simulink model "MoreElectricAircraftEMSHIL"  (R2023a)
settings: Solver=FixedStepAuto  StartTime=0.0  StopTime=350  RelTol=1e-3  EnableMultiTasking=on
PreLoadFcn:
  | Ts=100e-6;
InitFcn:
  | Ts=100e-6;
undefined symbols (not defined in the file): DiscIntNeverNeededParam, getfullname, IO682, Ion, Lithium
libraries: spsCurrentMeasurementLib x21, spsSeriesRLCBranchLib x19, spsVoltageMeasurementLib x19, speedgoatlib_IO682 x14, spsDiodeLib x10, spsControlledCurrentSourceLib x8, simulink x8, spsControlledVoltageSourceLib x7, spsIdealSwitchLib x6, spsThreePhaseParallelRLCLoadLib x1, spsPLL3phLib x1, spsThreePhaseVIMeasurementLib x1
(part 1 of 4)
settings Model: Creator=The MathWorks, Inc.  LastModifiedBy=steve.liu
settings SolverCC: ConcurrentTasks=on  AlgebraicLoopSolver=TrustRegion  PositivePriorityOrder=on  AutoInsertRateTranBlk=on
settings DataIOCC: LimitDataPoints=on  SaveFormat=Array  ReturnWorkspaceOutputs=off
settings OptimizationCC: BlockReduction=off  OptimizeBlockIOStorage=off  ReuseModelBlockBuffer=off  ExpressionDepthLimit=2147483647  EfficientMapNaN2IntZero=off
settings DebuggingCC: UnderspecifiedInitializationDetection=Classic  MergeDetectMultiDrivingBlocksExec=none  SolverPrmCheckMsg=warning  TasksWithSamePriorityMsg=none  UnconnectedInputMsg=warning  UnconnectedOutputMsg=warning  UnconnectedLineMsg=warning  AllowSymbolicDim=off  StateNameClashWarn=warning  PregeneratedLibrarySubsystemCodeDiagnostic=none  SFUnexpectedBacktrackingDiag=warning  SFNoUnconditionalDefaultTransitionDiag=warning  SFExecutionAtInitializationDiag=none  ArithmeticOperatorsInVariantConditions=warning
settings HardwareCC: ProdBitPerLong=64  ProdLongLongMode=on  ProdHWDeviceType=Intel->x86-64 (Linux 64)  TargetBitPerPointer=64  TargetBitPerSizeT=64  TargetBitPerPtrDiffT=64  TargetLongLongMode=on  TargetIntDivRoundTo=Zero  TargetEndianess=LittleEndian  TargetWordSize=64  TargetHWDeviceType=MATLAB Host
settings ModelReferenceCC: EnableRefExpFcnMdlSchedulingChecks=on  PropagateSignalLabelsOutOfModel=off
settings SFSimCC: SimUseLocalCustomCode=off  CustomCodeUndefinedFunction=UseInterfaceOnly
settings RTWCC: Description=Simulink Real-Time  SystemTargetFile=slrealtime.tlc  TemplateMakefile=slrealtime_default_tmf  RTWUseLocalCustomCode=off  Toolchain=Simulink Real-Time Toolchain  BuildConfiguration=Faster Runs  CodeExecutionProfiling=on  TargetLang=C++
settings CodeAppCC: MaxIdLength=128  StateflowObjectComments=on
settings ConfigComp: CovMetricSettings=dw  CovSaveCumulativeToWorkspaceVar=on  CovSaveSingleToWorkspaceVar=on  CovExternalEMLEnable=off  CovSFcnEnable=off
settings SimscapeCC: SimscapeNormalizeSystem=off

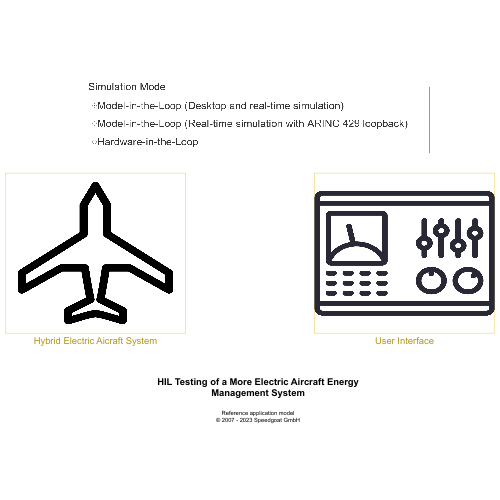
[thumbnail: Simulink's stored preview of the top-level diagram]
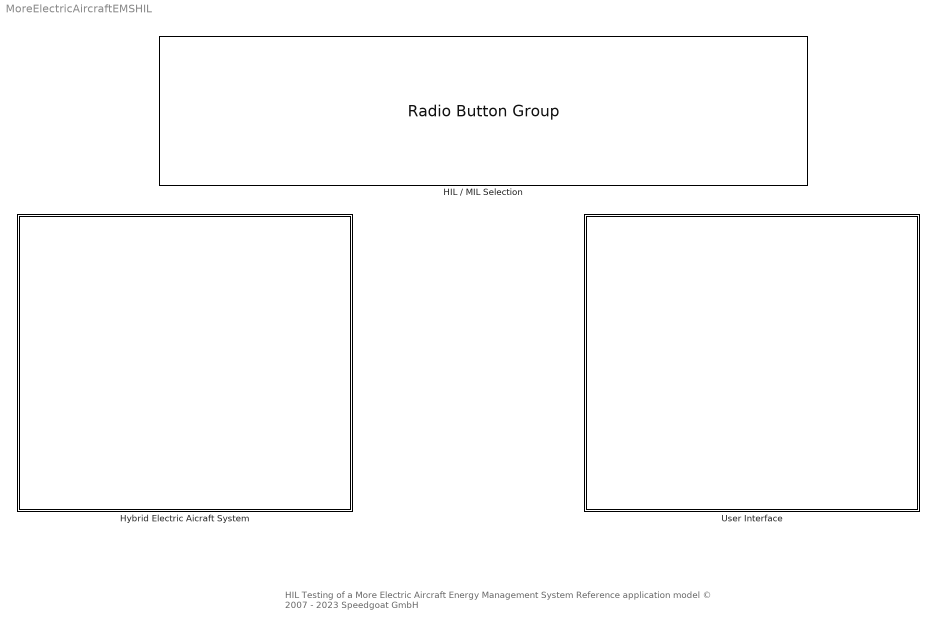
== system MoreElectricAircraftEMSHIL ==
  note: HIL Testing of a More Electric Aircraft Energy Management System
      |
      | Reference application model
      | © 2007 - 2023 Speedgoat GmbH
  HIL / MIL Selection : RadioButtonGroup  LabelPosition=Hide  SelectedLabel=Model-in-the-Loop (Desktop and real-time simulation)  ButtonGroupName=Simulation Mode
      settings: Values={{'Model-in-the-Loop (Desktop and real-time simulation)', 'Model-in-the-Loop (Real-time simulation with ARINC 429 loopback)', 'Hardware-in-the-Loop'}, [0 1 2]}
  Hybrid Electric Aicraft System : Subsystem
      mask Display: image('aircraft.png')
  User Interface : Subsystem
      mask Display: image('$imagefile'); % Use "Edit Image" on toolstrip to change.

== system MoreElectricAircraftEMSHIL/Hybrid Electric Aicraft System ==
  Energy Management System : Subsystem  Variant=on  VariantControl=Choice
      mask Display: image('$imagefile'); % Use "Edit Image" on toolstrip to change.
  Hybrid Electric Aicraft Plant : Subsystem
      mask Display: image('$imagefile'); % Use "Edit Image" on toolstrip to change.
  wires:
  Energy Management System/1(BusEMS) -> Hybrid Electric Aicraft Plant/1(In1)
  Hybrid Electric Aicraft Plant/1(Out4) -> Energy Management System/1(BusPlant)

== system MoreElectricAircraftEMSHIL/User Interface ==
  note: Power and Loads
      | [W]
  Aircraft Load(KVA) : SliderBlock  LabelPosition=Hide  ScaleMax=10
  Batt V : DisplayBlock  LabelPosition=Bottom  Format=Integer  Transparency=1
  Emergency Landing : ToggleSwitchBlock  LabelPosition=Hide
      settings: Values={{'Off', 'On'}, [0 1]}
  FC voltage V : DisplayBlock  LabelPosition=Bottom  Format=Integer  Transparency=1
  HIL Testing of a More Electric Aircraft Energy Management System : DashboardScope  TimeSpan=350  Ymin=-5000  Ymax=15000  ScaleAtStop=off  UpdateMode=Scroll
  Lamp : LampBlock  LabelPosition=Bottom
  Manual Load Control : ToggleSwitchBlock  LabelPosition=Hide
      settings: Values={{'Off', 'On'}, [0 1]}
  Oscilloscope : Subsystem
      mask Display: color('blue');disp('Instrumentation')
  SC V : DisplayBlock  LabelPosition=Bottom  Format=Integer  Transparency=1
  SOC (%) : DisplayBlock  LabelPosition=Bottom  Format=Integer  Transparency=1

== system MoreElectricAircraftEMSHIL/Hybrid Electric Aicraft System/Energy Management System ==
  BusPlant : Inport
  HIL : Subsystem  VariantControl=strcmp(get_param(getfullname(Simulink.findBlocks(bdroot,'Name','SimulationSelection')),'value'),'2')
  MIL : Subsystem  VariantControl=strcmp(get_param(getfullname(Simulink.findBlocks(bdroot,'Name','SimulationSelection')),'value'),'0')
  MIL-Loopback : Subsystem  VariantControl=strcmp(get_param(getfullname(Simulink.findBlocks(bdroot,'Name','SimulationSelection')),'value'),'1')
  BusEMS : Outport

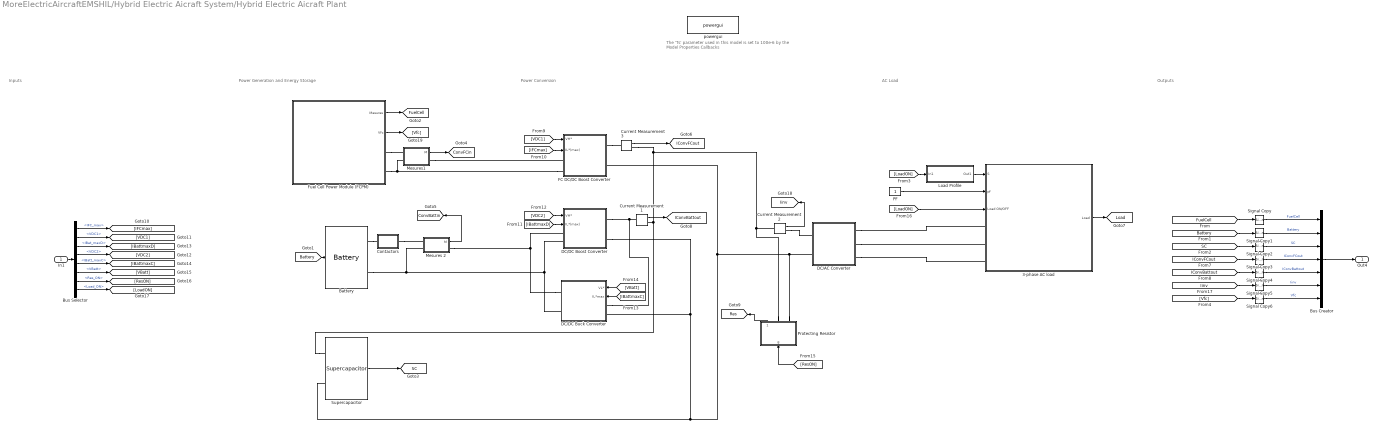
== system MoreElectricAircraftEMSHIL/Hybrid Electric Aicraft System/Hybrid Electric Aicraft Plant ==
  note: The 'Ts' parameter used in this model
      | is set to 100e-6  by the Model Properties Callbacks
  note: Power Generation and Energy Storage
  note: Power Conversion
  note: AC Load
  note: Inputs
  note: Outputs
  In1 : Inport
  3-phase AC load : Subsystem
      mask Display: image('load.png'); % Use "Edit Image" on toolstrip to change.
  Battery : spsBatteryLib/Battery  BatType=Lithium-Ion  ShowTempParam=off  ThermalPreset=no  ShowAgeParam=off  NomV=48  NomQ=40  SOC=65  Batt_Tr=20  PresetModel=off  MaxQ=40  MinV=36  FullV=55.8714  Dis_rate=17.3913  R=0.012  Normal_OP=36.1739  expZone="[52.3         1.96]"  current=[20 80]  Units=Ampere-hour  Tci=20  NomT=20  T2=-30  MaxQ2=4.8  FullV2=7.1  Normal_OP2=5.72  expZone2="[6.58  1]"  Rca=0.6  ti=1000  Dp=0  Neq0=0  Tsim=1e6  Ta1=25  Qeol=5.4*0.9  Reol=0.013333*1.2  Char_age=[2.3478, 3]  Dis_age=[2.3478, 10]  N1=1500  N2=10500  N3=1000  N4=1400  Ta2=45  N5=950
      settings: LibrarySourceBlock=electricdrivelib/Extra Sources/Battery
  Bus Creator : BusCreator  Inputs=7
  Bus Selector : BusSelector  OutputSignals=IFC_max,VDC1,IBat_maxD,VDC2,IBatt_maxC,VBatt,Res_ON,Load_ON
  Contactors : Subsystem
  Current Measurement1 : spsCurrentMeasurementLib/Current Measurement  PhasorSimulation=off  OutputType=Complex  PSBequivalent=0
  Current Measurement2 : spsCurrentMeasurementLib/Current Measurement  PhasorSimulation=off  OutputType=Complex  PSBequivalent=0
  Current Measurement3 : spsCurrentMeasurementLib/Current Measurement  PhasorSimulation=off  OutputType=Complex  PSBequivalent=0
  DC/AC Converter : Subsystem  mask(Average-value Inverter model){VL=200, f=400, n=97}
      mask prompts: VL "Output Line Voltage (Vrms)"; f "Output frequency (Hz)"; n "Nominal Efficiency (%)"
      mask help: This block represents an average-value inverter model which includes the converter efficiency.
      mask Display: image('inverter.png'); % Use "Edit Image" on toolstrip to change.
  DC/DC Boost Converter : Subsystem  mask(Average value DC/DC boost converter){Inom=18, n=[80 88], Tr=0.1, CL=15.6}
      mask prompts: Inom "Full load current (A)"; n "Efficiency @ Full and 10% load  (%) [n1, n2]"; Tr "Response time (s) (Voltage Regulator)"; CL "Load Capacitance (F)"
      mask help: This block implements an average-value DC/DC boost converter. Two inputs are provided for output voltage regulation and input current limitation
      mask Display: image('CCCCconverter.png'); % Use "Edit Image" on toolstrip to change.
  DC/DC Buck Converter : Subsystem  mask(Average Value Buck DC/DC Converter){Inom=20, n=[80 88], Tr=0.1, CL=100e-3}
      mask prompts: Inom "Full load current (A)"; n "Efficiency @ Full and 10% load (%) [n1, n2]"; Tr "Response Time (s) (Voltage Regulator)"; CL "Load Capacitance (F)"
      mask help: This block implements an average-value DC/DC buck converter. Two inputs are provided for output voltage regulation and output current limitation
      mask init:
      | L=10e-3; C=800e-6+CL;
      | thau_s=Tr;  %response time
      | %Current regulator
      | zetai=0.995;
      | thau_si=0.1/10; 
      | %zetawni=4.6/thau_si;
      | zetawni=(-log(0.05*sqrt(1-zetai^2)))/thau_si;
      | Kpi=2*L*zetawni;
      | wni=zetawni/zetai;
      | Kii=L*wni^2;
      | %Voltage regulator
      | zetav=0.995;
      | thau_sv=thau_s; %response time
      | %zetawnv=4.6/thau_sv;
      | zetawnv=(-log(0.05*sqrt(1-zetav^2)))/thau_sv;
      | Kpv=2*C*zetawnv;
      | wnv=zetawnv/zetav;
      | Kiv=C*wnv^2;
      | k=((n(1)/100)-(n(2)/100))/(Inom-(0.1*Inom));
      | k0=(n(1)/100)-k*Inom;
      mask DialogControl ParameterTabVar0 Prompt: Parameters
      mask Display: image('CCCCconverter.png'); % Use "Edit Image" on toolstrip to change.
  FC DC/DC Boost Converter : Subsystem  mask(Average value DC/DC boost converter){Inom=45, n=[85 90], Tr=0.1, CL=15.6}
      mask prompts: Inom "Full load current (A)"; n "Efficiency @ Full and 10% load  (%) [n1, n2]"; Tr "Response time (s) (Voltage Regulator)"; CL "Load Capacitance (F)"
      mask help: This block implements an average-value DC/DC boost converter. Two inputs are provided for output voltage regulation and input current limitation
      mask Display: image('CCCCconverter.png'); % Use "Edit Image" on toolstrip to change.
  Fuel Cell Power Module (FCPM) : Subsystem
      mask Display: image('FuelCell.png'); % Use "Edit Image" on toolstrip to change.
  Load Profile : Subsystem
      mask Display: image('$imagefile'); % Use "Edit Image" on toolstrip to change.
  Mesures 2 : Subsystem
  Mesures1 : Subsystem
  PF : Constant
  Protecting Resistor : Subsystem
      mask Display: image('resistor.png'); % Use "Edit Image" on toolstrip to change.
  Signal Copy{,1..6} (7 alike) : SignalConversion  OverrideOpt=off
  Supercapacitor : spsSupercapacitorLib/Supercapacitor  C=15.6  Rdc=150e-3  Voltage=291.6  Ns=108  Np=1  Vinit=270  Temp=25  PresetModel=on  EstParam=off  Nc=1  r=1e-9  epsilon=6.0208e-10  Ich=10  Vstern="[0.161  2.7  7.8]"  Self_dis=on  Ioc=10  Vself="[48  47.8  47.06  44.65]"  demandeplot=off  I="[10  20 100  500]"  Units=sec  Vmax=0  If=0  deltaV=0.3  alpha=0.3  sec=0
      settings: LibrarySourceBlock=electricdrivelib/Extra Sources/Supercapacitor
  powergui : spspowerguiLib/powergui  Priority=1  SimulationMode=Discrete  SampleTime=Ts  frequency=60  Iterations=50  frequencyindice=0  Pbase=100e6  ErrMax=1e-4  UnitsV=kV  UnitsW=MW  buscounter=0  FunctionMessages=off  echomessages=off  EnableUseOfTLC=off  CurrentSourceSwitches=off  DisableSnubberDevices=off  DisableRonSwitches=off  DisableVfSwitches=off  DisplayEquations=off  AutomaticDiscreteSolvers=off  SolverType=Tustin/Backward Euler (TBE)  Interpol=off  ExternalGateDelay=off  methode=off  Ts=0  x0status=blocks  SPID=off  SwTol=0  HookPort=off  NonlinearTolerance=1e-4  nMaxIteration=100  ContinueOnMaxIteration=off  RestoreLinks=warning  ResistiveCurrentMeasurement=off  Frange=[0:2:500]  Ylog=off  Xlog=on  ShowGrid=off  save=off  variable=ZData  structure=0  ZoomFFT=off  StartTime=0.0  cycles=1  DisplayStyle=1  fundamental=60  FreqAxis=off  MaxFrequency=1000  frequencyindicesteady=1  RmsSteady=1  display=off
  Out4 : Outport
  tag scope: Battery=global, ConvBattin=global, ConvFCin=global, FuelCell=global, IConvBattout=global, IConvFCout=global, Iinv=global, Load=global, Res=global, SC=global
  wires:
  Mesures1/1(M) -> [ConvFCin]
  [IBattmaxC] -> DC/DC Buck Converter/2(IL*max)
  [ResON] -> Protecting Resistor/1(g)
  [VDC1] -> FC DC/DC Boost Converter/1(VH*)
  [VDC2] -> DC/DC Boost Converter/1(VH*)
  Protecting Resistor/1(Mesures) -> [Res]
  [IFCmax] -> FC DC/DC Boost Converter/2(IL*(max))
  Mesures 2/1(M) -> [ConvBattin]
  [LoadON] -> 3-phase AC load/3(Load ON/OFF)
  [VBatt] -> DC/DC Buck Converter/1(VL*)
  Supercapacitor/1 -> [SC]
  PF/1 -> 3-phase AC load/2(pf)
  Fuel Cell Power Module (FCPM)/1(Mesures) -> [FuelCell]
  [IBattmaxD] -> DC/DC Boost Converter/2(IL*(max))
  Current Measurement3/1 -> [IConvFCout]
  3-phase AC load/1(Load) -> [Load]
  Battery/1 -> [Battery]
  Current Measurement2/1 -> [Iinv]
  Current Measurement1/1 -> [IConvBattout]
  [LoadON] -> Load Profile/1(In1)
  Load Profile/1(Out1) -> 3-phase AC load/1(S)
  [Battery] -> Signal Copy1/1
  [FuelCell] -> Signal Copy/1
  [SC] -> Signal Copy2/1
  [IConvFCout] -> Signal Copy3/1
  [IConvBattout] -> Signal Copy4/1
  [Iinv] -> Signal Copy5/1
  Signal Copy/1 -> Bus Creator/1  "FuelCell"
  Signal Copy1/1 -> Bus Creator/2  "Battery"
  Signal Copy2/1 -> Bus Creator/3  "SC"
  Signal Copy3/1 -> Bus Creator/4  "IConvFCout"
  Signal Copy4/1 -> Bus Creator/5  "IConvBattout"
  Signal Copy5/1 -> Bus Creator/6  "Iinv"
  Bus Creator/1 -> Out4/1
  In1/1 -> Bus Selector/1
  Bus Selector/1 -> [IFCmax]  "<IFC_max>"
  Bus Selector/2 -> [VDC1]  "<VDC1>"
  Bus Selector/3 -> [IBattmaxD]  "<IBat_maxD>"
  Bus Selector/4 -> [VDC2]  "<VDC2>"
  Bus Selector/5 -> [IBattmaxC]  "<IBatt_maxC>"
  Bus Selector/6 -> [VBatt]  "<VBatt>"
  Bus Selector/7 -> [ResON]  "<Res_ON>"
  Bus Selector/8 -> [LoadON]  "<Load_ON>"
  Fuel Cell Power Module (FCPM)/2(Vfc) -> [Vfc]
  [Vfc] -> Signal Copy6/1
  Signal Copy6/1 -> Bus Creator/7  "Vfc"
  connections:
  Battery/LConn1 -- Contactors/LConn1
  DC/DC Buck Converter/LConn1 -- DC/DC Boost Converter/RConn1 -- Current Measurement1/LConn1
  Mesures1/RConn1 -- FC DC/DC Boost Converter/LConn1
  Battery/LConn2 -- Mesures 2/LConn2 -- DC/DC Buck Converter/RConn2 -- DC/DC Boost Converter/LConn2
  FC DC/DC Boost Converter/RConn1 -- Current Measurement3/LConn1
  DC/AC Converter/RConn3 -- 3-phase AC load/LConn3
  Supercapacitor/LConn1 -- Current Measurement1/RConn1 -- Current Measurement3/RConn1 -- Protecting Resistor/RConn1 -- Current Measurement2/LConn1
  DC/DC Boost Converter/RConn2 -- DC/DC Buck Converter/LConn2 -- Supercapacitor/LConn2 -- Protecting Resistor/RConn2 -- DC/AC Converter/LConn2 -- FC DC/DC Boost Converter/RConn2
  FC DC/DC Boost Converter/LConn2 -- Mesures1/LConn2 -- Fuel Cell Power Module (FCPM)/RConn2
  DC/AC Converter/RConn1 -- 3-phase AC load/LConn1
  Fuel Cell Power Module (FCPM)/RConn1 -- Mesures1/LConn1
  DC/AC Converter/RConn2 -- 3-phase AC load/LConn2
  DC/DC Buck Converter/RConn1 -- Mesures 2/RConn1 -- DC/DC Boost Converter/LConn1
  Contactors/RConn1 -- Mesures 2/LConn1
  Current Measurement2/RConn1 -- DC/AC Converter/LConn1

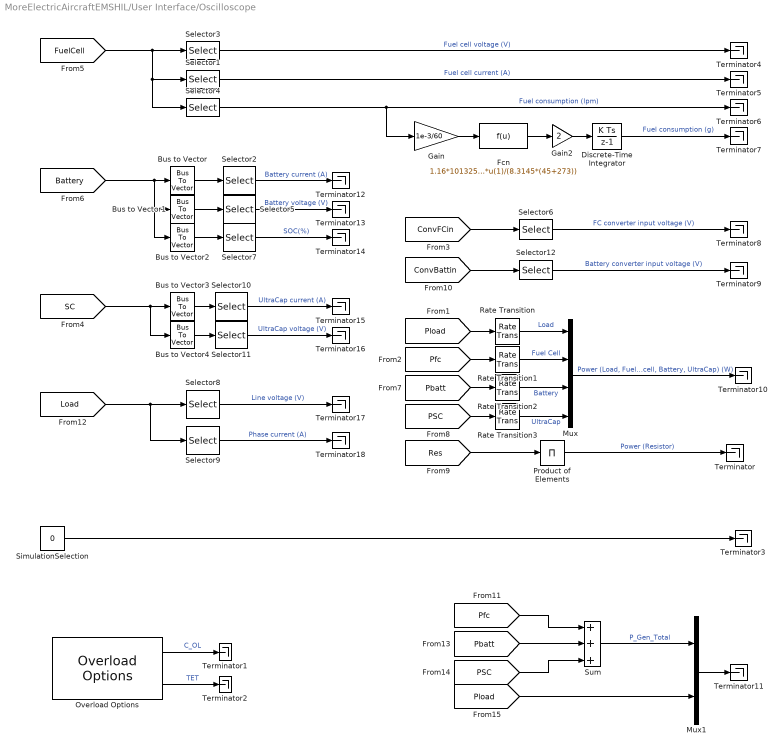
== system MoreElectricAircraftEMSHIL/User Interface/Oscilloscope ==
  Bus to Vector{,1..4} (5 alike) : BusToVector
  Discrete-Time Integrator : DiscreteIntegrator  SampleTime=Ts  ICPrevOutput=DiscIntNeverNeededParam  ICPrevScaledInput=DiscIntNeverNeededParam
  Fcn : Fcn  Expr=1.16*101325*u(1)/(8.3145*(45+273))
  Gain : Gain  Gain=1e-3/60
  Gain2 : Gain  Gain=2
  Mux : Mux
  Mux1 : Mux  Inputs=2
  Overload Options : slrealtimetgmanagement/Overload Options  startupDur=100  startupDurSrc=Tunable Parameter  maxOverload=100000  maxOverloadSrc=Tunable Parameter  TETFlag=on
  Product of Elements : Product  Inputs=*
  Rate Transition{,1..3} (4 alike) : RateTransition  OutPortSampleTime=0.01
  Selector1 : Selector  InputPortWidth=7  IndexOptions=Index vector (dialog)  Indices=3  OutputSizes=1
  Selector10 : Selector  InputPortWidth=3  IndexOptions=Index vector (dialog)  Indices=[1]  OutputSizes=1
  Selector11 : Selector  InputPortWidth=3  IndexOptions=Index vector (dialog)  Indices=[2]  OutputSizes=1
  Selector12 : Selector  InputPortWidth=2  IndexOptions=Index vector (dialog)  Indices=2  OutputSizes=1
  Selector2 : Selector  InputPortWidth=3  IndexOptions=Index vector (dialog)  Indices=[2]  OutputSizes=1
  Selector3 : Selector  InputPortWidth=7  IndexOptions=Index vector (dialog)  Indices=2  OutputSizes=1
  Selector4 : Selector  InputPortWidth=7  IndexOptions=Index vector (dialog)  Indices=5  OutputSizes=1
  Selector5 : Selector  InputPortWidth=3  IndexOptions=Index vector (dialog)  Indices=[3]  OutputSizes=1
  Selector6 : Selector  InputPortWidth=2  IndexOptions=Index vector (dialog)  Indices=2  OutputSizes=1
  Selector7 : Selector  InputPortWidth=3  IndexOptions=Index vector (dialog)  Indices=[1]  OutputSizes=1
  Selector8 : Selector  InputPortWidth=6  IndexOptions=Index vector (dialog)  Indices=[1]  OutputSizes=1
  Selector9 : Selector  InputPortWidth=6  IndexOptions=Index vector (dialog)  Indices=4  OutputSizes=1
  SimulationSelection : Constant  Value=0  OutDataTypeStr=uint8
  Sum : Sum  Inputs=+++
  Terminator{,1..18} (19 alike) : Terminator
  wires:
  Selector1/1 -> Terminator5/1  "Fuel cell current (A)"
  Selector3/1 -> Terminator4/1  "Fuel cell voltage (V)"
  [FuelCell] -> Selector3/1, Selector1/1, Selector4/1
  Selector5/1 -> Terminator13/1  "Battery voltage (V)"
  Selector2/1 -> Terminator12/1  "Battery current (A)"
  [Battery] -> Bus to Vector/1, Bus to Vector1/1, Bus to Vector2/1
  Selector11/1 -> Terminator16/1  "UltraCap voltage (V)"
  Selector10/1 -> Terminator15/1  "UltraCap current (A)"
  [SC] -> Bus to Vector4/1, Bus to Vector3/1
  Mux/1 -> Terminator10/1  "Power (Load, Fuel cell, Battery, UltraCap) (W)"
  Selector7/1 -> Terminator14/1  "SOC(%)"
  [Load] -> Selector9/1, Selector8/1
  Selector4/1 -> Terminator6/1, Gain/1  "Fuel consumption (lpm)"
  [Pload] -> Rate Transition/1
  [Pfc] -> Rate Transition1/1
  [Pbatt] -> Rate Transition2/1
  [PSC] -> Rate Transition3/1
  Gain/1 -> Fcn/1
  Fcn/1 -> Gain2/1
  Discrete-Time Integrator/1 -> Terminator7/1  "Fuel consumption (g)"
  Gain2/1 -> Discrete-Time Integrator/1
  Selector8/1 -> Terminator17/1  "Line voltage (V)"
  Selector9/1 -> Terminator18/1  "Phase current (A)"
  [ConvFCin] -> Selector6/1
  [ConvBattin] -> Selector12/1
  Selector6/1 -> Terminator8/1  "FC converter input voltage (V)"
  Selector12/1 -> Terminator9/1  "Battery converter input voltage (V)"
  Product of Elements/1 -> Terminator/1  "Power (Resistor)"
  [Res] -> Product of Elements/1
  Bus to Vector/1 -> Selector2/1
  Bus to Vector1/1 -> Selector5/1
  Bus to Vector2/1 -> Selector7/1
  Bus to Vector3/1 -> Selector10/1
  Bus to Vector4/1 -> Selector11/1
  Overload Options/2 -> Terminator2/1  "TET"
  Overload Options/1 -> Terminator1/1  "C_OL"
  Rate Transition/1 -> Mux/1  "Load"
  Rate Transition1/1 -> Mux/2  "Fuel Cell"
  Rate Transition2/1 -> Mux/3  "Battery"
  Rate Transition3/1 -> Mux/4  "UltraCap"
  Sum/1 -> Mux1/1  "P_Gen_Total"
  [Pload] -> Mux1/2
  Mux1/1 -> Terminator11/1
  [Pbatt] -> Sum/2
  [Pfc] -> Sum/1
  [PSC] -> Sum/3
  SimulationSelection/1 -> Terminator3/1

== system MoreElectricAircraftEMSHIL/Hybrid Electric Aicraft System/Energy Management System/HIL ==
  BusPlant : Inport
  Plant Rx : Subsystem  VariantControl=strcmp(get_param(getfullname(Simulink.findBlocks(bdroot,'Name','SimulationSelection')),'value'),'1')
      settings: PortSchema="{\"entries\":[{\"content\":{\"sides\":[{\"content\":{},\"type\":\"ConnectorPlacement.EquallySpacedRectSide\",\"uuid\":\"0c6f668b-a29c-42cd-bda6-91865cced16a\"},{\"content\":{\"side\":\"RIGHT\"},\"type\":\"ConnectorPlacement.EquallySpacedRectSide\",\"uuid\":\"7c419dc2-febf-4fba-9c42-2dac0ff32ed4\"},{\"content\":{\"connectorIds\":[\"Out1\"],\"side\":\"TOP\"},\"type\":\"ConnectorPlacement.EquallySpacedRectSide\",\"uuid\":\"f890f873-3c1e-481b-963a-d6b0448ae5f3\"}]},\"type\":\"ConnectorPlacement.EquallySpacedConnector\",\"uuid\":\"73046853-24ab-401a-be97-4c9da5376ff6\"}],\"packageUris\":[\"http://schema.mathworks.com/mf0/Connector/R2020b\"],\"version\":\"1.0\"}"
      mask Display: image('$imagefile'); % Use "Edit Image" on toolstrip to change.
  Plant Tx : Subsystem  VariantControl=strcmp(get_param(getfullname(Simulink.findBlocks(bdroot,'Name','SimulationSelection')),'value'),'1')
      settings: PortSchema="{\"entries\":[{\"content\":{\"sides\":[{\"content\":{},\"type\":\"ConnectorPlacement.EquallySpacedRectSide\",\"uuid\":\"ca674eb5-fb94-4202-b8d0-5664a17d79c3\"},{\"content\":{\"side\":\"RIGHT\"},\"type\":\"ConnectorPlacement.EquallySpacedRectSide\",\"uuid\":\"17984780-2d4e-48b0-8f73-31f6f9763c95\"},{\"content\":{\"side\":\"TOP\"},\"type\":\"ConnectorPlacement.EquallySpacedRectSide\",\"uuid\":\"c301ca29-45ff-4c1e-83fe-12dfababd426\"},{\"content\":{\"connectorIds\":[\"In1\"],\"side\":\"BOTTOM\"},\"type\":\"ConnectorPlacement.EquallySpacedRectSide\",\"uuid\":\"2f710d20-78f0-4498-bb85-d21ba6b27c93\"}]},\"type\":\"ConnectorPlacement.EquallySpacedConnector\",\"uuid\":\"1bf9fc79-8700-4a4a-8cdf-39255c72147f\"}],\"packageUris\":[\"http://schema.mathworks.com/mf0/Connector/R2020b\"],\"version\":\"1.0\"}"
      mask Display: image('$imagefile'); % Use "Edit Image" on toolstrip to change.
  BusEMS : Outport  VectorParamsAs1DForOutWhenUnconnected=off
  wires:
  BusPlant/1 -> Plant Tx/1(BusPlant)
  Plant Rx/1(BusEMS) -> BusEMS/1

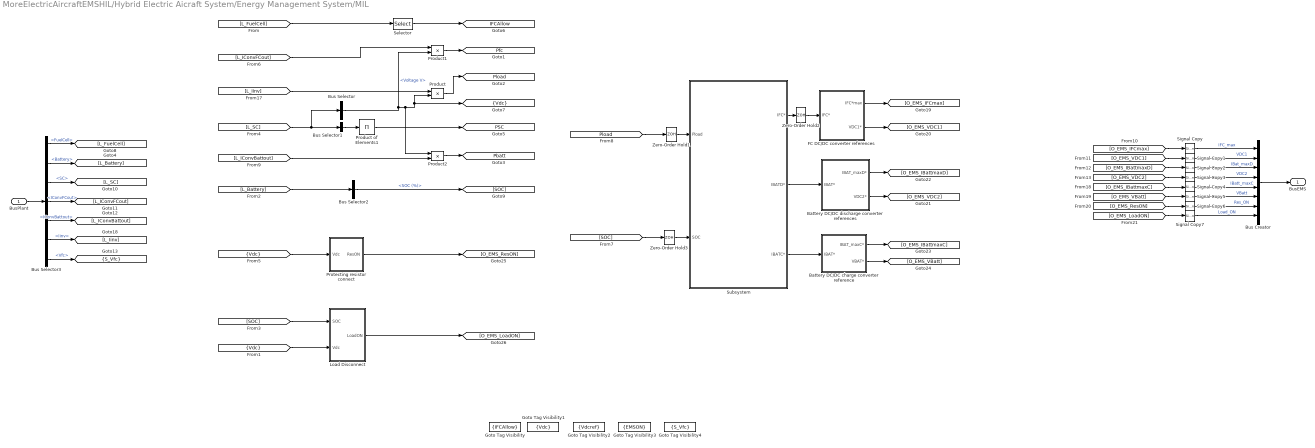
== system MoreElectricAircraftEMSHIL/Hybrid Electric Aicraft System/Energy Management System/MIL ==
  BusPlant : Inport
  Battery DC/DC charge converter reference : Subsystem
  "Battery DC/DC discharge converter references " : Subsystem
  Bus Creator : BusCreator  Inputs=8
  Bus Selector : BusSelector  OutputSignals=Voltage V
  Bus Selector1 : BusSelector  OutputSignals=Current I,Voltage V  OutputAsBus=on
  Bus Selector2 : BusSelector  OutputSignals=SOC (%)
  Bus Selector3 : BusSelector  OutputSignals=FuelCell,Battery,SC,IConvFCout,IConvBattout,Iinv,Vfc
  FC DC/DC converter references : Subsystem
  Goto Tag Visibility : GotoTagVisibility  GotoTag=IFCAllow
  Goto Tag Visibility1 : GotoTagVisibility  GotoTag=Vdc
  Goto Tag Visibility2 : GotoTagVisibility  GotoTag=Vdcref
  Goto Tag Visibility3 : GotoTagVisibility  GotoTag=EMSON
  Goto Tag Visibility4 : GotoTagVisibility  GotoTag=S_Vfc
  Load Disconnect : Subsystem
  Product : Product  RndMeth=Zero
  Product of Elements1 : Product  Inputs=*
  Product1 : Product  RndMeth=Zero
  Product2 : Product  RndMeth=Zero
  Protecting resistor connect : Subsystem
  Selector : Selector  InputPortWidth=7  IndexOptions=Index vector (dialog)  Indices=1  OutputSizes=1
  Signal Copy{,1..7} (8 alike) : SignalConversion  OverrideOpt=off
  Subsystem : Subsystem
  Zero-Order Hold1 : ZeroOrderHold  SampleTime=200e-3
  Zero-Order Hold2 : ZeroOrderHold  SampleTime=200e-3
  Zero-Order Hold3 : ZeroOrderHold  SampleTime=200e-3
  BusEMS : Outport  VectorParamsAs1DForOutWhenUnconnected=off
  tag scope: IFCAllow=global, PSC=global, Pbatt=global, Pfc=global, Pload=global, S_Vfc=scoped, Vdc=scoped
  wires:
  Bus Selector/1 -> Product1/2, Product2/1, Product/2, [Vdc]  "<Voltage V>"
  [L_IConvFCout] -> Product1/1
  [L_IConvBattout] -> Product2/2
  [L_Iinv] -> Product/1
  [L_SC] -> Bus Selector/1, Bus Selector1/1
  Product/1 -> [Pload]
  Product1/1 -> [Pfc]
  Product2/1 -> [Pbatt]
  Bus Selector1/1 -> Product of Elements1/1
  Product of Elements1/1 -> [PSC]
  Selector/1 -> [IFCAllow]
  [L_Battery] -> Bus Selector2/1
  Bus Selector2/1 -> [SOC]  "<SOC (%)>"
  [SOC] -> Load Disconnect/1(SOC)
  [Vdc] -> Load Disconnect/2(Vdc)
  [Vdc] -> Protecting resistor connect/1(Vdc)
  Subsystem/1(IFC*) -> Zero-Order Hold2/1
  [Pload] -> Zero-Order Hold1/1
  [SOC] -> Zero-Order Hold3/1
  Zero-Order Hold2/1 -> FC DC/DC converter references/1(IFC*)
  Subsystem/2(IBATD*) -> "Battery DC/DC discharge converter references "/1(IBAT*)
  Subsystem/3(IBATC*) -> Battery DC/DC charge converter reference/1(IBAT*)
  Zero-Order Hold1/1 -> Subsystem/1(Pload)
  Zero-Order Hold3/1 -> Subsystem/2(SOC)
  FC DC/DC converter references/1(IFC*max) -> [O_EMS_IFCmax]
  FC DC/DC converter references/2(VDC1*) -> [O_EMS_VDC1]
  "Battery DC/DC discharge converter references "/1(IBAT_maxD*) -> [O_EMS_IBattmaxD]
  "Battery DC/DC discharge converter references "/2(VDC2*) -> [O_EMS_VDC2]
  Battery DC/DC charge converter reference/1(IBAT_maxC*) -> [O_EMS_IBattmaxC]
  Battery DC/DC charge converter reference/2(VBAT*) -> [O_EMS_VBatt]
  Protecting resistor connect/1(ResON) -> [O_EMS_ResON]
  Load Disconnect/1(LoadON) -> [O_EMS_LoadON]
  BusPlant/1 -> Bus Selector3/1
  Bus Selector3/1 -> [L_FuelCell]  "<FuelCell>"
  Bus Selector3/2 -> [L_Battery]  "<Battery>"
  Bus Selector3/3 -> [L_SC]  "<SC>"
  Bus Selector3/4 -> [L_IConvFCout]  "<IConvFCout>"
  Bus Selector3/5 -> [L_IConvBattout]  "<IConvBattout>"
  Bus Selector3/6 -> [L_Iinv]  "<Iinv>"
  [L_FuelCell] -> Selector/1
  [O_EMS_IFCmax] -> Signal Copy/1
  [O_EMS_VDC1] -> Signal Copy1/1
  [O_EMS_IBattmaxD] -> Signal Copy2/1
  [O_EMS_VDC2] -> Signal Copy3/1
  [O_EMS_IBattmaxC] -> Signal Copy4/1
  [O_EMS_VBatt] -> Signal Copy5/1
  [O_EMS_ResON] -> Signal Copy6/1
  [O_EMS_LoadON] -> Signal Copy7/1
  Signal Copy1/1 -> Bus Creator/2  "VDC1"
  Signal Copy2/1 -> Bus Creator/3  "IBat_maxD"
  Signal Copy3/1 -> Bus Creator/4  "VDC2"
  Signal Copy4/1 -> Bus Creator/5  "IBatt_maxC"
  Signal Copy5/1 -> Bus Creator/6  "VBatt"
  Signal Copy6/1 -> Bus Creator/7  "Res_ON"
  Signal Copy7/1 -> Bus Creator/8  "Load_ON"
  Signal Copy/1 -> Bus Creator/1  "IFC_max"
  Bus Creator/1 -> BusEMS/1
  Bus Selector3/7 -> [S_Vfc]  "<Vfc>"

== system MoreElectricAircraftEMSHIL/Hybrid Electric Aicraft System/Energy Management System/MIL-Loopback ==
  BusPlant : Inport
  EMS : Subsystem  VariantControl=strcmp(get_param(getfullname(Simulink.findBlocks(bdroot,'Name','SimulationSelection')),'value'),'0')
      mask Display: image('$imagefile'); % Use "Edit Image" on toolstrip to change.
  EMS Rx : Subsystem  VariantControl=strcmp(get_param(getfullname(Simulink.findBlocks(bdroot,'Name','SimulationSelection')),'value'),'1')
      settings: PortSchema="{\"entries\":[{\"content\":{\"sides\":[{\"content\":{},\"type\":\"ConnectorPlacement.EquallySpacedRectSide\",\"uuid\":\"e292a2d6-b746-4d3a-991b-06f84f221c80\"},{\"content\":{\"side\":\"RIGHT\"},\"type\":\"ConnectorPlacement.EquallySpacedRectSide\",\"uuid\":\"f08863f0-9241-4871-b41a-1d1d2ed46e21\"},{\"content\":{\"side\":\"TOP\"},\"type\":\"ConnectorPlacement.EquallySpacedRectSide\",\"uuid\":\"e540036f-aa38-4866-ab92-cec750947e09\"},{\"content\":{\"connectorIds\":[\"Out1\"],\"side\":\"BOTTOM\"},\"type\":\"ConnectorPlacement.EquallySpacedRectSide\",\"uuid\":\"8bfbe013-9f95-4eb9-9c1d-013b23463782\"}]},\"type\":\"ConnectorPlacement.EquallySpacedConnector\",\"uuid\":\"57c2ad21-b109-4500-9c54-46aeabef525e\"}],\"packageUris\":[\"http://schema.mathworks.com/mf0/Connector/R2020b\"],\"version\":\"1.0\"}"
      mask Display: image('$imagefile'); % Use "Edit Image" on toolstrip to change.
  EMS Tx : Subsystem  VariantControl=strcmp(get_param(getfullname(Simulink.findBlocks(bdroot,'Name','SimulationSelection')),'value'),'1')
      settings: PortSchema="{\"entries\":[{\"content\":{\"sides\":[{\"content\":{},\"type\":\"ConnectorPlacement.EquallySpacedRectSide\",\"uuid\":\"65f07a85-8c21-40c2-bbb0-85dcd72c1f04\"},{\"content\":{\"side\":\"RIGHT\"},\"type\":\"ConnectorPlacement.EquallySpacedRectSide\",\"uuid\":\"fa93bd10-5dbc-449b-aa5e-07593847a8a6\"},{\"content\":{\"connectorIds\":[\"In1\"],\"side\":\"TOP\"},\"type\":\"ConnectorPlacement.EquallySpacedRectSide\",\"uuid\":\"9c469b41-bab3-4394-8bbc-3c7bad027204\"}]},\"type\":\"ConnectorPlacement.EquallySpacedConnector\",\"uuid\":\"8402933d-3e19-4874-8a16-1518d29b091a\"}],\"packageUris\":[\"http://schema.mathworks.com/mf0/Connector/R2020b\"],\"version\":\"1.0\"}"
      mask Display: image('$imagefile'); % Use "Edit Image" on toolstrip to change.
  Plant Rx : Subsystem  VariantControl=strcmp(get_param(getfullname(Simulink.findBlocks(bdroot,'Name','SimulationSelection')),'value'),'1')
      settings: PortSchema="{\"entries\":[{\"content\":{\"sides\":[{\"content\":{},\"type\":\"ConnectorPlacement.EquallySpacedRectSide\",\"uuid\":\"0c6f668b-a29c-42cd-bda6-91865cced16a\"},{\"content\":{\"side\":\"RIGHT\"},\"type\":\"ConnectorPlacement.EquallySpacedRectSide\",\"uuid\":\"7c419dc2-febf-4fba-9c42-2dac0ff32ed4\"},{\"content\":{\"connectorIds\":[\"Out1\"],\"side\":\"TOP\"},\"type\":\"ConnectorPlacement.EquallySpacedRectSide\",\"uuid\":\"f890f873-3c1e-481b-963a-d6b0448ae5f3\"}]},\"type\":\"ConnectorPlacement.EquallySpacedConnector\",\"uuid\":\"73046853-24ab-401a-be97-4c9da5376ff6\"}],\"packageUris\":[\"http://schema.mathworks.com/mf0/Connector/R2020b\"],\"version\":\"1.0\"}"
      mask Display: image('$imagefile'); % Use "Edit Image" on toolstrip to change.
  Plant Tx : Subsystem  VariantControl=strcmp(get_param(getfullname(Simulink.findBlocks(bdroot,'Name','SimulationSelection')),'value'),'1')
      settings: PortSchema="{\"entries\":[{\"content\":{\"sides\":[{\"content\":{},\"type\":\"ConnectorPlacement.EquallySpacedRectSide\",\"uuid\":\"ca674eb5-fb94-4202-b8d0-5664a17d79c3\"},{\"content\":{\"side\":\"RIGHT\"},\"type\":\"ConnectorPlacement.EquallySpacedRectSide\",\"uuid\":\"17984780-2d4e-48b0-8f73-31f6f9763c95\"},{\"content\":{\"side\":\"TOP\"},\"type\":\"ConnectorPlacement.EquallySpacedRectSide\",\"uuid\":\"c301ca29-45ff-4c1e-83fe-12dfababd426\"},{\"content\":{\"connectorIds\":[\"In1\"],\"side\":\"BOTTOM\"},\"type\":\"ConnectorPlacement.EquallySpacedRectSide\",\"uuid\":\"2f710d20-78f0-4498-bb85-d21ba6b27c93\"}]},\"type\":\"ConnectorPlacement.EquallySpacedConnector\",\"uuid\":\"1bf9fc79-8700-4a4a-8cdf-39255c72147f\"}],\"packageUris\":[\"http://schema.mathworks.com/mf0/Connector/R2020b\"],\"version\":\"1.0\"}"
      mask Display: image('$imagefile'); % Use "Edit Image" on toolstrip to change.
  BusEMS : Outport  VectorParamsAs1DForOutWhenUnconnected=off
  wires:
  EMS Rx/1(Out1) -> EMS/1(BusPlant)
  BusPlant/1 -> Plant Tx/1(BusPlant)
  EMS/1(BusEMS) -> EMS Tx/1(IFC*max1)
  Plant Rx/1(BusEMS) -> BusEMS/1

== system MoreElectricAircraftEMSHIL/Hybrid Electric Aicraft System/Hybrid Electric Aicraft Plant/3-phase AC load ==
  S : Inport
  pf : Inport  Port=2
  Load ON/OFF : Inport  Port=3
  1 kW 0.5 kvar @ 208V3 : spsThreePhaseParallelRLCLoadLib/Three-Phase Parallel RLC Load  LConnTagsString=A|B|C  Configuration=Y (grounded)  NominalVoltage=200  Vabc=[1e3 1e3 1e3]  Vabcp=[1e3 1e3 1e3]  NominalFrequency=400  UnbalancedPower=off  ActivePower=1e-6  InductivePower=0  CapacitivePower=0  Pabc=[10e3 9e3 11e3]  QLabc=[100 90 110]  QCabc=[100 90 110]  Pabcp=[10e3 9e3 11e3]  QLabcp=[100 90 110]  QCabcp=[100 90 110]  Measurements=None  LoadType=constant Z
  Complex to Real-Imag : ComplexToRealImag
  Controlled Current Source : spsControlledCurrentSourceLib/Controlled Current Source  Initialize=off  Source_Type=AC  Amplitude=0  Phase=0  Frequency=0  Measurements=None
  Controlled Current Source1 : spsControlledCurrentSourceLib/Controlled Current Source  Initialize=off  Source_Type=AC  Amplitude=0  Phase=0  Frequency=0  Measurements=None
  Demux : Demux  Outputs=3
  Demux1 : Demux  Outputs=2
  Divide2 : Product  Inputs=/*
  Dynamic Impedance : Subsystem
  Gain : Gain  Gain=1/3
  Ground : Ground
  Mux1 : Mux  Inputs=3
  Mux2 : Mux  Inputs=2
  PLL (3ph) : spsPLL3phLib/PLL (3ph)  Fmin=390  Par_Init=[0, 60]  ParK=[180, 3200, 1]  TcD=1e-4  MaxRateChangeFreq=12  FilterCutOffFreq=25  Ts=0  AGC=on
  Product : Product  RndMeth=Zero
  Real-Imag to Complex : RealImagToComplex
  Saturation : Saturate  UpperLimit=1  LowerLimit=0.001
  Saturation1 : Saturate  UpperLimit=1  LowerLimit=-1
  Saturation2 : Saturate  UpperLimit=inf  LowerLimit=0.001
  Selector : Selector  InputPortWidth=3  IndexOptions=Index vector (dialog)  Indices=[1 2]  OutputSizes=1
  Terminator1 : Terminator
  Terminator2 : Terminator
  Three-Phase V-I Measurement1 : spsThreePhaseVIMeasurementLib/Three-Phase V-I Measurement  VoltageMeasurement=phase-to-ground  SetLabelV=off  LabelV=Vabc  Vpu=off  VpuLL=off  CurrentMeasurement=yes  SetLabelI=off  LabelI=Iabc  Ipu=off  Pbase=100e6  Vbase=500e3  OutputType=Complex  PhasorSimulation=off  PSBequivalent=0
  Unit Delay : UnitDelay  SampleTime=Ts  HasFrameUpgradeWarning=on
  Unit Delay1 : UnitDelay  SampleTime=Ts  HasFrameUpgradeWarning=on
  abc to dq0 : spsabctodq0Lib/abc to dq0  Alignment=90 degrees behind phase A axis
  dq0 to abc : spsdq0toabcLib/dq0 to abc  Alignment=90 degrees behind phase A axis
  A : PMIOPort  Side=Left
  B : PMIOPort  Port=2  Side=Left
  C : PMIOPort  Port=3  Side=Left
  Load : Outport  VectorParamsAs1DForOutWhenUnconnected=off
  wires:
  Divide2/1 -> Complex to Real-Imag/1
  Dynamic Impedance/1(Z) -> Divide2/1
  Three-Phase V-I Measurement1/1 -> PLL (3ph)/1, abc to dq0/1, Mux2/1
  Demux/3 -> Terminator1/1
  Mux1/1 -> dq0 to abc/1
  Ground/1 -> Mux1/3
  Complex to Real-Imag/2 -> Mux1/2
  Complex to Real-Imag/1 -> Mux1/1
  Real-Imag to Complex/1 -> Divide2/2
  Demux/2 -> Real-Imag to Complex/2
  Demux/1 -> Real-Imag to Complex/1
  S/1 -> Saturation2/1
  Selector/1 -> Demux1/1
  Demux1/1 -> Unit Delay/1
  Demux1/2 -> Unit Delay1/1
  pf/1 -> Saturation1/1
  Gain/1 -> Dynamic Impedance/1(S)
  Unit Delay/1 -> Controlled Current Source/1
  Unit Delay1/1 -> Controlled Current Source1/1
  Three-Phase V-I Measurement1/2 -> Mux2/2
  Mux2/1 -> Load/1
  Saturation/1 -> Product/2
  Load ON/OFF/1 -> Saturation/1
  Product/1 -> Gain/1
  Saturation1/1 -> Dynamic Impedance/2(pf)
  Saturation2/1 -> Product/1
  PLL (3ph)/2 -> abc to dq0/2, dq0 to abc/2
  abc to dq0/1 -> Demux/1
  PLL (3ph)/1 -> Terminator2/1
  dq0 to abc/1 -> Selector/1
  connections:
  C/RConn1 -- Three-Phase V-I Measurement1/LConn3 -- 1 kW 0.5 kvar @ 208V3/LConn3
  Three-Phase V-I Measurement1/LConn2 -- B/RConn1 -- 1 kW 0.5 kvar @ 208V3/LConn2
  Three-Phase V-I Measurement1/LConn1 -- A/RConn1 -- 1 kW 0.5 kvar @ 208V3/LConn1
  Controlled Current Source1/LConn1 -- Three-Phase V-I Measurement1/RConn2
  Controlled Current Source/RConn1 -- Three-Phase V-I Measurement1/RConn3 -- Controlled Current Source1/RConn1
  Controlled Current Source/LConn1 -- Three-Phase V-I Measurement1/RConn1

== system MoreElectricAircraftEMSHIL/Hybrid Electric Aicraft System/Hybrid Electric Aicraft Plant/Contactors ==
  Compare To Zero : simulink/Logic and Bit Operations/Compare To Zero  relop=>  OutDataTypeStr=boolean
  Current Measurement : spsCurrentMeasurementLib/Current Measurement  PhasorSimulation=off  OutputType=Complex  PSBequivalent=0
  Ideal Switch : spsIdealSwitchLib/Ideal Switch  Ron=0.001  Lon=0  IC=0  Rs=1e5  Cs=inf  Measurements=off
  Series RLC Branch : spsSeriesRLCBranchLib/Series RLC Branch  LConnTagsString=__new0  RConnTagsString=__new0  BranchType=R  Resistance=0.175  Inductance=1e-3  SetiL0=off  InitialCurrent=0  Capacitance=1e-6  Setx0=off  InitialVoltage=0  Measurements=None
  Series RLC Branch1 : spsSeriesRLCBranchLib/Series RLC Branch  LConnTagsString=__new0  RConnTagsString=__new0  BranchType=R  Resistance=0.07  Inductance=1e-3  SetiL0=off  InitialCurrent=0  Capacitance=1e-6  Setx0=off  InitialVoltage=0  Measurements=None
  A : PMIOPort  Side=Left
  B : PMIOPort  Port=2  Side=Right
  wires:
  Current Measurement/1 -> Compare To Zero/1
  Compare To Zero/1 -> Ideal Switch/1
  connections:
  Ideal Switch/LConn1 -- Series RLC Branch/LConn1 -- Current Measurement/RConn1
  A/RConn1 -- Current Measurement/LConn1
  Ideal Switch/RConn1 -- Series RLC Branch1/LConn1
  Series RLC Branch1/RConn1 -- B/RConn1 -- Series RLC Branch/RConn1

== system MoreElectricAircraftEMSHIL/Hybrid Electric Aicraft System/Hybrid Electric Aicraft Plant/DC//AC Converter ==
  Add : Sum  Inputs=+-
  Control open loop1 : Subsystem
  Controlled Current Source : spsControlledCurrentSourceLib/Controlled Current Source  Initialize=on  Source_Type=AC  Amplitude=0  Phase=0  Frequency=0  Measurements=None
  Controlled Voltage Source : spsControlledVoltageSourceLib/Controlled Voltage Source  Initialize=on  Source_Type=AC  Amplitude=0  Phase=0  Frequency=0  Measurements=None
  Controlled Voltage Source1 : spsControlledVoltageSourceLib/Controlled Voltage Source  Initialize=on  Source_Type=AC  Amplitude=0  Phase=0  Frequency=0  Measurements=None
  Current Measurement : spsCurrentMeasurementLib/Current Measurement  PhasorSimulation=off  OutputType=Complex  PSBequivalent=0
  Current Measurement2 : spsCurrentMeasurementLib/Current Measurement  PhasorSimulation=off  OutputType=Complex  PSBequivalent=0
  Divide : Product  Inputs=*/
  Gain1 : Gain  Gain=n/100
  Product : Product  RndMeth=Zero
  Product1 : Product  RndMeth=Zero
  Saturation : Saturate  UpperLimit=inf  LowerLimit=0.01
  Selector : Selector  InputPortWidth=3  IndexOptions=Index vector (dialog)  Indices=1  OutputSizes=1
  Selector1 : Selector  InputPortWidth=3  IndexOptions=Index vector (dialog)  Indices=2  OutputSizes=1
  Unit Delay : UnitDelay  SampleTime=Ts  HasFrameUpgradeWarning=on
  Vab-inv1 : spsVoltageMeasurementLib/Voltage Measurement  Tag=PoWeRsYsTeMmEaSuReMeNt  PhasorSimulation=off  OutputType=Magnitude  PSBequivalent=0
  Vab-inv2 : spsVoltageMeasurementLib/Voltage Measurement  Tag=PoWeRsYsTeMmEaSuReMeNt  PhasorSimulation=off  OutputType=Magnitude  PSBequivalent=0
  Vab-inv4 : spsVoltageMeasurementLib/Voltage Measurement  Tag=PoWeRsYsTeMmEaSuReMeNt  PhasorSimulation=off  OutputType=Magnitude  PSBequivalent=0
  A : PMIOPort  Side=Right
  +Vdc : PMIOPort  Port=2  Side=Left
  B : PMIOPort  Port=3  Side=Right
  -Vdc : PMIOPort  Port=4  Side=Left
  C : PMIOPort  Port=5  Side=Right
  wires:
  Vab-inv1/1 -> Product/2
  Current Measurement/1 -> Product/1
  Product/1 -> Add/1
  Vab-inv2/1 -> Product1/1
  Current Measurement2/1 -> Product1/2
  Product1/1 -> Add/2
  Add/1 -> Divide/1
  Vab-inv4/1 -> Gain1/1
  Saturation/1 -> Divide/2
  Divide/1 -> Unit Delay/1
  Control open loop1/1(g) -> Selector/1, Selector1/1
  Selector/1 -> Controlled Voltage Source/1
  Selector1/1 -> Controlled Voltage Source1/1
  Gain1/1 -> Saturation/1
  Unit Delay/1 -> Controlled Current Source/1
  connections:
  -Vdc/RConn1 -- Vab-inv4/LConn2 -- Controlled Current Source/RConn1
  Controlled Voltage Source/LConn1 -- Controlled Voltage Source1/RConn1 -- Vab-inv1/LConn2 -- Vab-inv2/LConn1 -- B/RConn1
  Controlled Voltage Source/RConn1 -- Vab-inv1/LConn1 -- Current Measurement/LConn1
  Controlled Voltage Source1/LConn1 -- Vab-inv2/LConn2 -- Current Measurement2/LConn1
  A/RConn1 -- Current Measurement/RConn1
  C/RConn1 -- Current Measurement2/RConn1
  +Vdc/RConn1 -- Controlled Current Source/LConn1 -- Vab-inv4/LConn1

== system MoreElectricAircraftEMSHIL/Hybrid Electric Aicraft System/Hybrid Electric Aicraft Plant/DC//DC Boost Converter ==
  VH* : Inport
  IL*(max) : Inport  Port=2
  Constant : Constant  Value=60
  DC/DC Boost Converter : Subsystem  mask(Average Value Boost DC/DC Converter){Inom=Inom, n=n, Tr=Tr, CL=CL}
      mask prompts: Inom "Full load current (A)"; n "Efficiency at Full and 10% load (%) [n1, n2]"; Tr "Response Time (s) (Voltage Regulator)"; CL "Load Capacitance (F)"
      mask help: This block implements an average-value DC/DC boost converter. Two inputs are provided for output voltage regulation and input current limitation
      mask init:
      | L=100e-6; C=800e-6+CL;
      | thau_s=Tr;  % response time
      | %Current regulator
      | zetai=0.707;
      | thau_si=0.1/10; 
      | %zetawni=4.6/thau_si;
      | zetawni=(-log(0.05*sqrt(1-zetai^2)))/thau_si;
      | Kpi=2*L*zetawni;
      | wni=zetawni/zetai;
      | Kii=L*wni^2;
      | %Voltage regulator
      | zetav=0.707;
      | thau_sv=thau_s; %response time
      | %zetawnv=4.6/thau_sv;
      | zetawnv=(-log(0.05*sqrt(1-zetav^2)))/thau_sv;
      | Kpv=2*C*zetawnv;
      | wnv=zetawnv/zetav;
      | Kiv=C*wnv^2;
      | k=((n(1)/100)-(n(2)/100))/(Inom-(0.1*Inom));
      | k0=(n(1)/100)-k*Inom;
      mask DialogControl ParameterTabVar0 Prompt: Parameters
  DC/DC Buck Converter For DC bus precharge : Subsystem  mask(Average Value Buck DC/DC Converter){Inom=0.88*Inom, n=n, Tr=Tr, CL=CL}
      mask prompts: Inom "Full oad current (A)"; n "Efficiency @ Full and 10% load (%) [n1, n2]"; Tr "Response Time (s) (Voltage Regulator)"; CL "Load Capacitance (F)"
      mask help: This block implements an average-value DC/DC buck converter. Two inputs are provided for output voltage regulation and output current limitation
      mask init:
      | L=100e-6; C=800e-6+CL;
      | thau_s=Tr;  %response time
      | %Current regulator
      | zetai=0.707;
      | thau_si=0.1/10; 
      | %zetawni=4.6/thau_si;
      | zetawni=(-log(0.05*sqrt(1-zetai^2)))/thau_si;
      | Kpi=2*L*zetawni;
      | wni=zetawni/zetai;
      | Kii=L*wni^2;
      | %Voltage regulator
      | zetav=0.707;
      | thau_sv=thau_s; %response time
      | %zetawnv=4.6/thau_sv;
      | zetawnv=(-log(0.05*sqrt(1-zetav^2)))/thau_sv;
      | Kpv=2*C*zetawnv;
      | wnv=zetawnv/zetav;
      | Kiv=C*wnv^2;
      | k=((n(1)/100)-(n(2)/100))/(Inom-(0.1*Inom));
      | k0=(n(1)/100)-k*Inom;
      mask DialogControl ParameterTabVar0 Prompt: Parameters
  +VH : PMIOPort  Side=Right
  +VL : PMIOPort  Port=2  Side=Left
  -VH : PMIOPort  Port=3  Side=Right
  -VL : PMIOPort  Port=4  Side=Left
  wires:
  IL*(max)/1 -> DC/DC Boost Converter/2(IL*(max))
  VH*/1 -> DC/DC Boost Converter/1(VH*)
  Constant/1 -> DC/DC Buck Converter For DC bus precharge/1(VL*)
  DC/DC Buck Converter For DC bus precharge/1(Iinbuck) -> [Iinbuck]
  [Iinbuck] -> DC/DC Boost Converter/3(Iinbuck)
  connections:
  DC/DC Boost Converter/RConn1 -- +VH/RConn1 -- DC/DC Buck Converter For DC bus precharge/RConn1
  DC/DC Boost Converter/LConn1 -- +VL/RConn1 -- DC/DC Buck Converter For DC bus precharge/LConn1
  DC/DC Boost Converter/LConn2 -- -VL/RConn1 -- DC/DC Buck Converter For DC bus precharge/LConn2
  DC/DC Buck Converter For DC bus precharge/RConn2 -- -VH/RConn1 -- DC/DC Boost Converter/RConn2

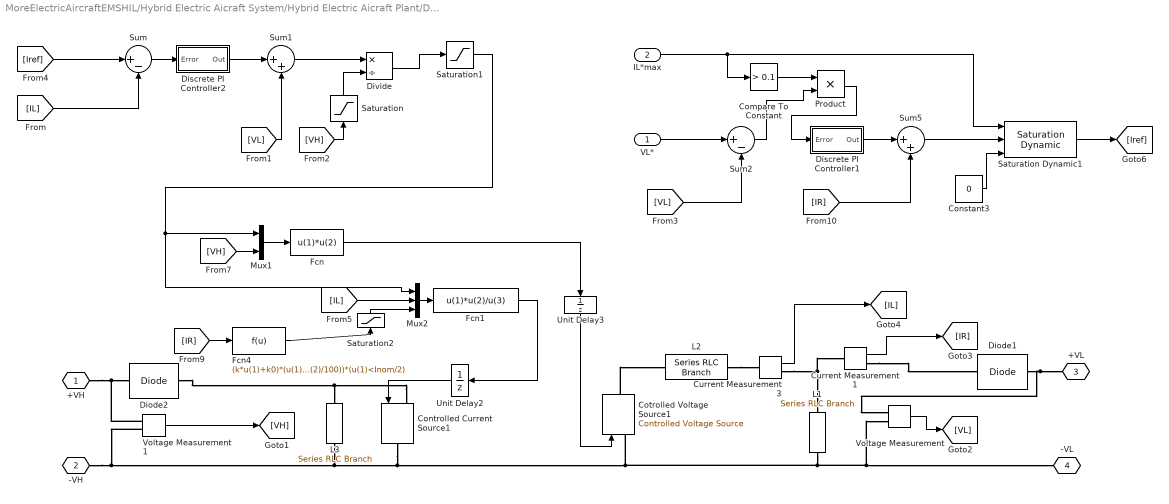
== system MoreElectricAircraftEMSHIL/Hybrid Electric Aicraft System/Hybrid Electric Aicraft Plant/DC//DC Buck Converter ==
  VL* : Inport
  IL*max : Inport  Port=2
  Compare To Constant : simulink/Logic and Bit Operations/Compare To Constant  relop=>  const=0.1  OutDataTypeStr=uint8
  Constant3 : Constant  Value=0
  Controlled Current Source1 : spsControlledCurrentSourceLib/Controlled Current Source  Initialize=on  Source_Type=DC  Amplitude=0  Phase=0  Frequency=0  Measurements=None
  Cotrolled Voltage Source1 : spsControlledVoltageSourceLib/Controlled Voltage Source  Initialize=on  Source_Type=DC  Amplitude=0  Phase=0  Frequency=0  Measurements=None
  Current Measurement1 : spsCurrentMeasurementLib/Current Measurement  PhasorSimulation=off  OutputType=Complex  PSBequivalent=0
  Current Measurement3 : spsCurrentMeasurementLib/Current Measurement  PhasorSimulation=off  OutputType=Complex  PSBequivalent=0
  Diode1 : spsDiodeLib/Diode  Ron=0.001  Lon=0  Vf=0  IC=0  UseSnubber=off  Rs=1e6  Cs=250e-9  Measurements=off
  Diode2 : spsDiodeLib/Diode  Ron=0.001  Lon=0  Vf=0  IC=0  UseSnubber=off  Rs=1e6  Cs=250e-9  Measurements=off
  Discrete PI Controller1 : Subsystem  DialogController=POWERSYS.PowerSysDialog  mask(Discrete PI Controller){Kp=Kpv, Ki=Kiv, Par_Limits=[1 -1], Init=0, Ts=Ts}
      mask prompts: Kp "Proportional gain (Kp):"; Ki "Integral gain (Ki):"; Par_Limits "Output limits: [ Upper   Lower ]"; Init "Output initial value:"; Ts "Sample time:"
      mask help: This block implements a discrete PI controller.
      mask init:
      | UpperLimit=Par_Limits(1);
      | LowerLimit=Par_Limits(2);
      | power_initmask();
      mask Help: This block is part of a subset of blocks in the Extras library that does not have documentation associated with it, other than the block mask description.
      mask Display: disp('PI');
  Discrete PI Controller2 : Subsystem  DialogController=POWERSYS.PowerSysDialog  mask(Discrete PI Controller){Kp=Kpi, Ki=Kii, Par_Limits=[1 -1], Init=0, Ts=Ts}
      mask prompts: Kp "Proportional gain (Kp):"; Ki "Integral gain (Ki):"; Par_Limits "Output limits: [ Upper   Lower ]"; Init "Output initial value:"; Ts "Sample time:"
      mask help: This block implements a discrete PI controller.
      mask init:
      | UpperLimit=Par_Limits(1);
      | LowerLimit=Par_Limits(2);
      | power_initmask();
      mask Help: This block is part of a subset of blocks in the Extras library that does not have documentation associated with it, other than the block mask description.
      mask Display: disp('PI');
  Divide : Product  Inputs=*/  SampleTime=Ts
  Fcn : Fcn  Expr=u(1)*u(2)
  Fcn1 : Fcn  Expr=u(1)*u(2)/u(3)
  Fcn4 : Fcn  Expr=(k*u(1)+k0)*(u(1)>=Inom/2)+((n(2)/100))*(u(1)<Inom/2)  SampleTime=Ts
  L1 : spsSeriesRLCBranchLib/Series RLC Branch  LConnTagsString=__new0  RConnTagsString=__new0  BranchType=RC  Resistance=0.01  Inductance=10e-6  SetiL0=off  InitialCurrent=100  Capacitance=800e-6  Setx0=off  InitialVoltage=0  Measurements=None
  L2 : spsSeriesRLCBranchLib/Series RLC Branch  LConnTagsString=__new0  RConnTagsString=__new0  BranchType=L  Resistance=0.3  Inductance=L  SetiL0=off  InitialCurrent=100  Capacitance=100e-6  Setx0=off  InitialVoltage=0  Measurements=None
  L3 : spsSeriesRLCBranchLib/Series RLC Branch  LConnTagsString=__new0  RConnTagsString=__new0  BranchType=R  Resistance=2e6  Inductance=10e-6  SetiL0=off  InitialCurrent=100  Capacitance=800e-6  Setx0=off  InitialVoltage=0  Measurements=None
  Mux1 : Mux  Inputs=2
  Mux2 : Mux  Inputs=3
  Product : Product  RndMeth=Zero
  Saturation : Saturate  UpperLimit=inf  LowerLimit=0.001  SampleTime=Ts
  Saturation Dynamic1 : simulink/Discontinuities/Saturation Dynamic  OutMin=[]  OutMax=[]  OutDataTypeStr=Inherit: Same as second input  OutDataType=fixdt(1, 16)  OutScaling=2^-10  DoSatur=off
  Saturation1 : Saturate  UpperLimit=1  LowerLimit=0  SampleTime=Ts
  Saturation2 : Saturate  UpperLimit=inf  LowerLimit=0.001  SampleTime=Ts
  Sum : Sum  Inputs=|+-
  Sum1 : Sum  Inputs=|++
  Sum2 : Sum  Inputs=|+-
  Sum5 : Sum  Inputs=|++
  Unit Delay2 : UnitDelay  SampleTime=Ts  HasFrameUpgradeWarning=on
  Unit Delay3 : UnitDelay  SampleTime=Ts  HasFrameUpgradeWarning=on
  Voltage Measurement : spsVoltageMeasurementLib/Voltage Measurement  PhasorSimulation=off  OutputType=Complex  PSBequivalent=0
  Voltage Measurement1 : spsVoltageMeasurementLib/Voltage Measurement  PhasorSimulation=off  OutputType=Complex  PSBequivalent=0
  +VH : PMIOPort  Tag=PMCPort  Side=Left
  -VH : PMIOPort  Tag=PMCPort  Port=2  Side=Left
  +VL : PMIOPort  Tag=PMCPort  Port=3  Side=Right
  -VL : PMIOPort  Tag=PMCPort  Port=4  Side=Right
  wires:
  Mux2/1 -> Fcn1/1
  Mux1/1 -> Fcn/1
  Voltage Measurement/1 -> [VL]
  Voltage Measurement1/1 -> [VH]
  Current Measurement1/1 -> [IR]
  [IL] -> Mux2/2
  [VH] -> Mux1/2
  Fcn/1 -> Unit Delay3/1
  Fcn1/1 -> Unit Delay2/1
  [IL] -> Sum/2
  Sum/1 -> Discrete PI Controller2/1(Error)
  Discrete PI Controller2/1(Out) -> Sum1/1
  [VL] -> Sum1/2
  Sum1/1 -> Divide/1
  [VH] -> Saturation/1
  Saturation/1 -> Divide/2
  Divide/1 -> Saturation1/1
  Saturation1/1 -> Mux2/1, Mux1/1
  Sum2/1 -> Product/2
  Discrete PI Controller1/1(Out) -> Sum5/1
  Sum5/1 -> Saturation Dynamic1/2
  Constant3/1 -> Saturation Dynamic1/3
  Saturation Dynamic1/1 -> [Iref]
  Current Measurement3/1 -> [IL]
  [VL] -> Sum2/2
  [Iref] -> Sum/1
  IL*max/1 -> Saturation Dynamic1/1, Compare To Constant/1
  [IR] -> Fcn4/1
  VL*/1 -> Sum2/1
  Compare To Constant/1 -> Product/1
  Product/1 -> Discrete PI Controller1/1(Error)
  Saturation2/1 -> Mux2/3
  Fcn4/1 -> Saturation2/1
  [IR] -> Sum5/2
  Unit Delay2/1 -> Controlled Current Source1/1
  Unit Delay3/1 -> Cotrolled Voltage Source1/1
  connections:
  Voltage Measurement1/LConn2 -- -VH/RConn1 -- Cotrolled Voltage Source1/LConn1 -- -VL/RConn1 -- Voltage Measurement/LConn2 -- L1/RConn1 -- Controlled Current Source1/RConn1 -- L3/RConn1
  Voltage Measurement1/LConn1 -- Diode2/LConn1 -- +VH/RConn1
  Cotrolled Voltage Source1/RConn1 -- L2/RConn1
  Current Measurement3/RConn1 -- Current Measurement1/LConn1 -- L1/LConn1
  Current Measurement1/RConn1 -- Diode1/LConn1
  Diode1/RConn1 -- Voltage Measurement/LConn1 -- +VL/RConn1
  Controlled Current Source1/LConn1 -- Diode2/RConn1 -- L3/LConn1
  L2/LConn1 -- Current Measurement3/LConn1
